simulink model "exp11_f2"  (R2020a)
settings: Solver=FixedStepAuto  StartTime=0.0  StopTime=5  FixedStep=0.01  RelTol=1e-3
settings Model: Creator=zengw  LastModifiedBy=zengw

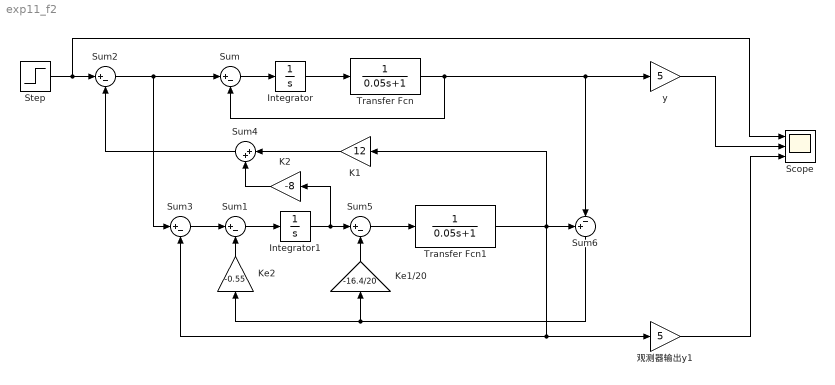
== system exp11_f2 ==
  Integrator : Integrator
  Integrator1 : Integrator  InitialCondition=0.02
  K1 : Gain  Gain=12
  K2 : Gain  Gain=-8
  Ke1/20 : Gain  Gain=-16.4/20
  Ke2 : Gain  Gain=-0.55
  Scope : Scope  NumInputPorts=3
  Step : Step  Time=0  SampleTime=0
  Sum{,1..3,5} (5 alike) : Sum  Inputs=|+-
  Sum4 : Sum  Inputs=|++
  Sum6 : Sum  Inputs=+-|
  Transfer Fcn : TransferFcn  Denominator=[0.05 1]
  Transfer Fcn1 : TransferFcn  Denominator=[0.05 1]
  y : Gain  Gain=5
  观测器输出y1 : Gain  Gain=5
  wires:
  Sum/1 -> Integrator/1
  Integrator/1 -> Transfer Fcn/1
  Transfer Fcn/1 -> y/1, Sum6/2, Sum/2
  Sum1/1 -> Integrator1/1
  Integrator1/1 -> Sum5/1, K2/1
  Transfer Fcn1/1 -> K1/1, Sum3/2, 观测器输出y1/1, Sum6/1
  K2/1 -> Sum4/2
  K1/1 -> Sum4/1
  Sum4/1 -> Sum2/2
  Step/1 -> Sum2/1, Scope/1
  Sum3/1 -> Sum1/1
  Ke2/1 -> Sum1/2
  Sum6/1 -> Ke2/1, Ke1/20/1
  y/1 -> Scope/2
  观测器输出y1/1 -> Scope/3
  Sum2/1 -> Sum3/1, Sum/1
  Sum5/1 -> Transfer Fcn1/1
  Ke1/20/1 -> Sum5/2
